simulink library "gyro_calibration_algorithm_atomic_sub_chart_library"  (R2014b)
settings: Solver=ode45  StartTime=0.0  StopTime=10.0  RelTol=1e-3
libraries: legonxtlib x1
settings Model: Creator=mbiesiad  LastModifiedBy=gatinc

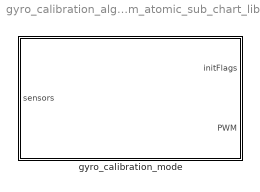
== system gyro_calibration_algorithm_atomic_sub_chart_library ==
  gyro_calibration_mode : Stateflow chart  TreatAsAtomicUnit=on  DSMNames=current_task_operation_status  DSMValues=current_mode_status

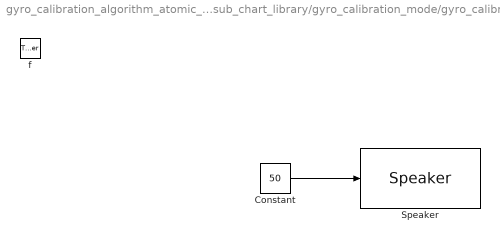
== system gyro_calibration_algorithm_atomic_sub_chart_library/gyro_calibration_mode/gyro_calibration_mode.GyroCalibration.Speak ==
  f : TriggerPort  TriggerType=function-call
      settings: CopyFcn=Stateflow.SLINSF.SimulinkMan.removeBlockPreDeleteFcn  PreDeleteFcn=Stateflow.SLINSF.SimulinkMan.unsafePredeleteFcn
  Constant : Constant  Value=50
  Speaker : legonxtlib/Speaker  sinputMode=Volume only  sspeakerFreq=800  sspeakerVolume=50  sspeakerDuration=100  blockPlatform=LegoMindstormsNXT
  wires:
  Constant/1 -> Speaker/1

== stateflow chart gyro_calibration_algorithm_atomic_sub_chart_library/gyro_calibration_mode ==
  state gyro_calibration_mode
    state GyroCalibration
      entry:
      desired_tail = single(0);
      during, exit:
      PWM.tail = tail_controller(sensors.theta_T,desired_tail);
      state Waiting
      state MoveTailDown
        entry:
        StatusLCD(uint16(100));
        during:
        desired_tail = desired_tail + single(0.0075);
      state StartCalibration
        entry:
        StatusLCD(uint16(101));
        initFlags.gyroInit = single(1);
        initFlags.gyroReset = single(1);
        initFlags.theta = single(1);
      state Wait
        entry: Speak;
      state MakeNoise
        during: Speak;
      state StartCalibration1
        entry:
        StatusLCD(uint16(102));
        initFlags.gyroInit = single(0);
        initFlags.gyroReset = single(0);
        initFlags.theta = single(0);
      state CalibComplete
        entry:
        StatusLCD(uint16(103));
        current_task_operation_status = OperationModeStatusEnum.SUCCESSFULLY_COMPLETED;
      state Speak [function] [commented out]
      (default) -> MoveTailDown
      Waiting -> gyro_calibration_mode.GyroCalibration.StartCalibration : after(1,sec)
      MoveTailDown -> gyro_calibration_mode.GyroCalibration.StartCalibration : [desired_tail >= single(1.85) ]
      gyro_calibration_mode.GyroCalibration.StartCalibration -> Wait : [sensors.touch]{Speak;}
      Wait -> MakeNoise : after(5,sec)
      MakeNoise -> StartCalibration1 : after(0.5,sec)
      StartCalibration1 -> CalibComplete
    state StartCalibration
    (default) -> gyro_calibration_mode.StartCalibration
    gyro_calibration_mode.StartCalibration -> GyroCalibration : [sensors.touch]
  data: current_task_operation_status data_store_memory; sensors input Bus: Sensors_Bus size=1; initFlags output Bus: Init_Bus size=1; PWM output Bus: PWM_bus size=1; desired_tail local
